simulink model "Tanques_otra_forma"  (R2021a)
settings: Solver=VariableStepAuto  StartTime=0.0  StopTime=20  RelTol=1e-3
settings Model: Creator=Santiago  LastModifiedBy=Santiago

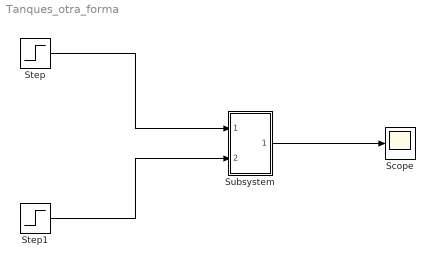
== system Tanques_otra_forma ==
  Scope : Scope
  Step : Step  SampleTime=0
  Step1 : Step  Time=10  SampleTime=0
  Subsystem : Subsystem
  wires:
  Step/1 -> Subsystem/1(In1)
  Step1/1 -> Subsystem/2(In2)
  Subsystem/1(Out1) -> Scope/1

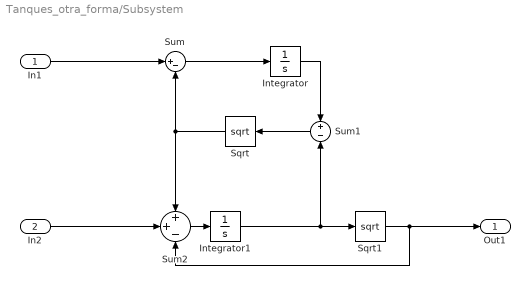
== system Tanques_otra_forma/Subsystem ==
  In1 : Inport
  In2 : Inport  Port=2
  Integrator : Integrator
  Integrator1 : Integrator
  Sqrt : Sqrt  SaturateOnIntegerOverflow=on
  Sqrt1 : Sqrt  SaturateOnIntegerOverflow=on
  Sum : Sum  Inputs=|+-
  Sum1 : Sum  Inputs=+|-
  Sum2 : Sum  Inputs=++-
  Out1 : Outport
  wires:
  In2/1 -> Sum2/2
  Sum2/1 -> Integrator1/1
  Integrator/1 -> Sum1/1
  Sum/1 -> Integrator/1
  Sqrt1/1 -> Out1/1, Sum2/3
  Sqrt/1 -> Sum/2, Sum2/1
  Integrator1/1 -> Sqrt1/1, Sum1/2
  Sum1/1 -> Sqrt/1
  In1/1 -> Sum/1
